simulink model "leggedRobotSim3DRig"  (R2026a)
settings: Solver=VariableStepAuto  StopTime=12  AbsTol=1e-3  EnableMultiTasking=on
values from neighbouring files (symbols this model uses):
  db = database()    [LeggedRobotSim.m]    (also in dbFunc.m; parameterSweep.m; parameterSweepDims.m)
  m = db.dims.m    [LeggedRobotSim.m]    (also in parameterSweep.m = db.dims.m_1 + db.dims.m_2 + 0.486; parameterSweepDims.m = db.dims.m_1 + db.dims.m_2 + 0.486)
  N = length(E)    [LeggedRobotSim.m]    (also in parameterSweep.m; parameterSweepDims.m)
undefined symbols (not defined in the file or in its folder): X, Y, Z
libraries: sm_lib x45, nesl_utility x15
(part 2 of 2)

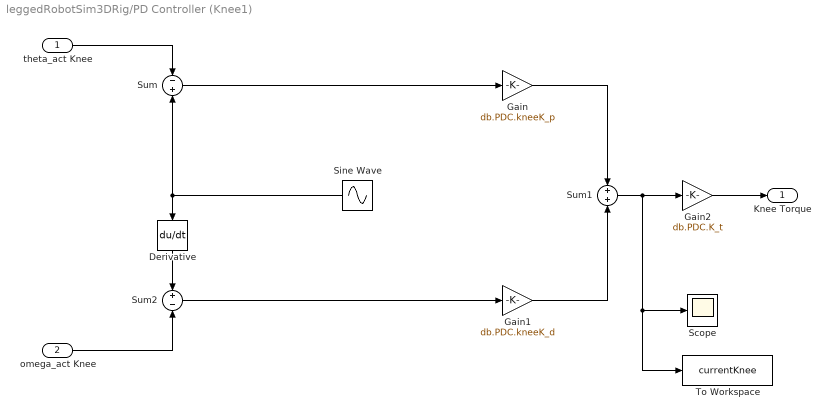
== system leggedRobotSim3DRig/PD Controller (Knee1) ==
  theta_act Knee : Inport
  omega_act Knee : Inport  Port=2
  Derivative : Derivative
  Gain : Gain  Gain=db.PDC.kneeK_p
  Gain1 : Gain  Gain=db.PDC.kneeK_d
  Gain2 : Gain  Gain=db.PDC.K_t
  Scope : Scope
      settings: ActiveDisplayYMinimum=-1  ActiveDisplayYMaximum=1  DataLoggingVariableName=ScopeData2
  Sine Wave : Sin  Amplitude=db.gait.theta_amp(2)  Frequency=db.gait.f_knee  Phase=db.gait.phi_knee1  SampleTime=0
  Sum : Sum  Inputs=-|+
  Sum1 : Sum  Inputs=+|+
  Sum2 : Sum  Inputs=+|-
  To Workspace : ToWorkspace  VariableName=currentKnee  SaveFormat=Timeseries  SampleTime=-1
  Knee Torque : Outport
  wires:
  Gain/1 -> Sum1/1
  theta_act Knee/1 -> Sum/1
  Sum/1 -> Gain/1
  Gain1/1 -> Sum1/2
  Gain2/1 -> Knee Torque/1
  Sum1/1 -> Gain2/1, To Workspace/1, Scope/1
  Sine Wave/1 -> Derivative/1, Sum/2
  Derivative/1 -> Sum2/1
  omega_act Knee/1 -> Sum2/2
  Sum2/1 -> Gain1/1

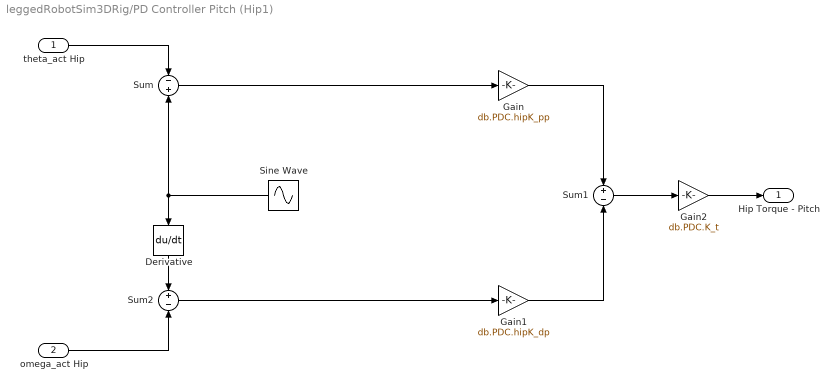
== system leggedRobotSim3DRig/PD Controller Pitch (Hip1) ==
  theta_act Hip : Inport
  omega_act Hip : Inport  Port=2
  Derivative : Derivative
  Gain : Gain  Gain=db.PDC.hipK_pp
  Gain1 : Gain  Gain=db.PDC.hipK_dp
  Gain2 : Gain  Gain=db.PDC.K_t
  Sine Wave : Sin  Amplitude=db.gait.theta_amp(1)  Frequency=db.gait.f_hip  Phase=db.gait.phi_hip1  SampleTime=0
  Sum : Sum  Inputs=-|+
  Sum1 : Sum  Inputs=+|-
  Sum2 : Sum  Inputs=+|-
  Hip Torque - Pitch : Outport
  wires:
  Sum1/1 -> Gain2/1
  Gain/1 -> Sum1/1
  theta_act Hip/1 -> Sum/1
  Sum/1 -> Gain/1
  Gain1/1 -> Sum1/2
  Gain2/1 -> Hip Torque - Pitch/1
  Sine Wave/1 -> Sum/2, Derivative/1
  Derivative/1 -> Sum2/1
  Sum2/1 -> Gain1/1
  omega_act Hip/1 -> Sum2/2

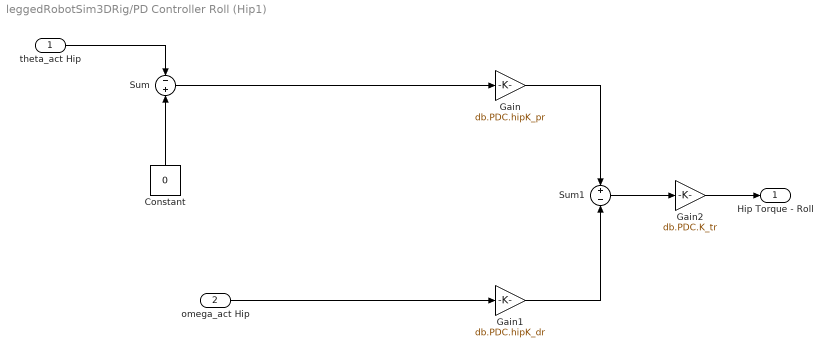
== system leggedRobotSim3DRig/PD Controller Roll (Hip1) ==
  theta_act Hip : Inport
  omega_act Hip : Inport  Port=2
  Constant : Constant  Value=0
  Gain : Gain  Gain=db.PDC.hipK_pr
  Gain1 : Gain  Gain=db.PDC.hipK_dr
  Gain2 : Gain  Gain=db.PDC.K_tr
  Sum : Sum  Inputs=-|+
  Sum1 : Sum  Inputs=+|-
  Hip Torque - Roll : Outport
  wires:
  Sum1/1 -> Gain2/1
  Gain/1 -> Sum1/1
  theta_act Hip/1 -> Sum/1
  Sum/1 -> Gain/1
  Gain1/1 -> Sum1/2
  Gain2/1 -> Hip Torque - Roll/1
  omega_act Hip/1 -> Gain1/1
  Constant/1 -> Sum/2
